simulink model "OPENXWD"  (R2022b)
settings: Solver=ode45  StartTime=0.0  StopTime=inf  RelTol=1e-3  EnableMultiTasking=on
PreLoadFcn:
  | run('Parameters\FSE_Parameters.m')
model workspace (MAT data in the model file):
  socvcb : containers.Map (value not decoded)
undefined symbols (not defined in the file): i_Diff
libraries: CarMaker4SL x21, simulink x16, eeGeneralControl x6
(part 3 of 8)

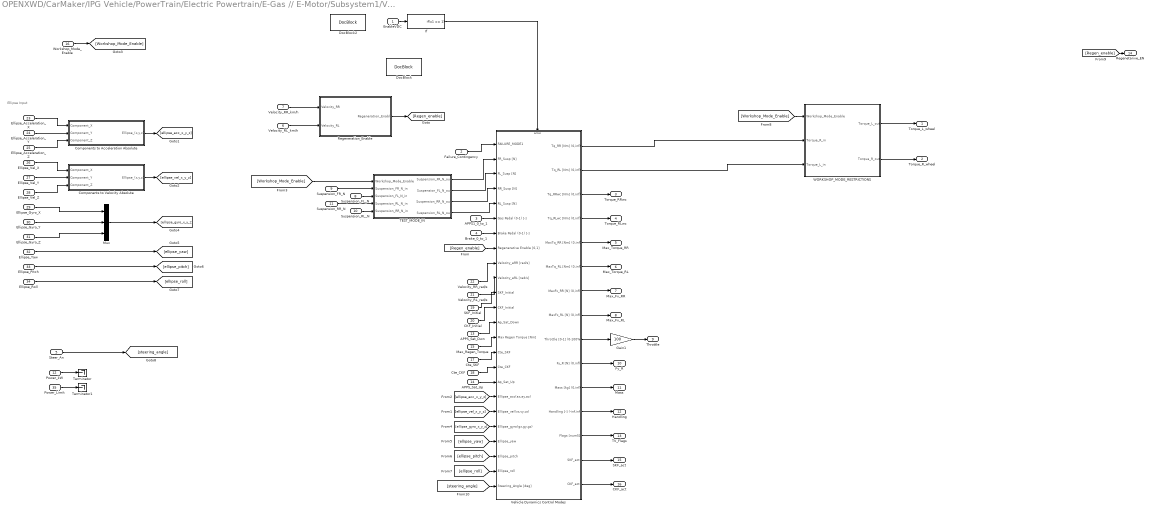
== system OPENXWD/CarMaker/IPG Vehicle/PowerTrain/Electric Powertrain/E-Gas // E-Motor/Subsystem1/VDC ==
  note: Ellipse Input
  EnableVDC : Inport
  Failure_Contingency : Inport  Port=2
  APPS1_0_to_1 : Inport  Port=3
  Brake_0_to_1 : Inport  Port=4
  Steer_An : Inport  Port=5
  Velocity_RL_km/h : Inport  Port=6
  Velocity_RR_km/h : Inport  Port=7
  Suspension_FL_N : Inport  Port=8
  Suspension_FR_N : Inport  Port=9
  Suspension_RL_N : Inport  Port=10
  Suspension_RR_N : Inport  Port=11
  Power_kW : Inport  Port=12
  APPS_Sat_Dwn : Inport  Port=13
  APPS_Sat_Up : Inport  Port=14
  Max_Regen_Torque : Inport  Port=15
  Workshop_Mode_Enable : Inport  Port=16
  Cte_SKF : Inport  Port=17
  Cte_CKF : Inport  Port=18
  SKF_Initial : Inport  Port=19
  CKF_Initial : Inport  Port=20
  Velocity_RL_rad/s : Inport  Port=21
  Velocity_RR_rad/s : Inport  Port=22
  Ellipse_Acceleration_X : Inport  Port=23
  Ellipse_Acceleration_Y : Inport  Port=24
  Ellipse_Acceleration_Z : Inport  Port=25
  Ellipse_Vel_X : Inport  Port=26
  Ellipse_Vel_Y : Inport  Port=27
  Ellipse_Vel_Z : Inport  Port=28
  Ellipse_Gyro_X : Inport  Port=29
  Ellipse_Gyro_Y : Inport  Port=30
  Ellipse_Gyro_Z : Inport  Port=31
  Ellipse_Yaw : Inport  Port=32
  Ellipse_Pitch : Inport  Port=33
  Ellipse_Roll : Inport  Port=34
  Power_Limit : Inport  Port=35
  Components to Acceleration Absolute : Subsystem
  Components to Velocity Absolute : Subsystem
  DocBlock : simulink/Model-Wide Utilities/DocBlock  DocumentType=Text
      content=|
      | This port activates the different modes that the VDC must be in according
      | to the signals that the Main ECU has available.
      |
      | Port Must be 1 to activate VDC 2018 Complete (Green)
      | Requirement: All sensors are connected (Ellipse, Steering, SuspensionRear
      | [SuspensionFront only needed to calculate Mass]).
      |
      | Port Must be 2 to activate VDC without Longitudinal (Yellow)
      | Requirement: No steering sensor data
      |
      | Port Must be 3 to activate Steering TV 2017 without TC (Orange)
      | Requirement: (No Ellipse) or (No SuspensionRear Data)
      |
      | Port Must be 4 to activate Rigid Axle (Red)
      | Requirement: (No Steering Sensor) and (No Ellipse or No SuspensionRear)
  DocBlock2 : simulink/Model-Wide Utilities/DocBlock  DocumentType=Text
      content=|
      | Enable Vehicle Dynamics Control.
      |
      | This port must be 1 if the calculations for VDC must be made
  Gain1 : Gain  Gain=100
  If : If  IfExpression=u1 == 1  ShowElse=off
  Mux : Mux  Inputs=3
  Regeneration_Enable : Subsystem  TreatAsAtomicUnit=on
  TEST_MODE_IN : Subsystem  TreatAsAtomicUnit=on
  Terminator : Terminator
  Terminator1 : Terminator
  Vehicle Dynamics Control Modes : Subsystem
  WORKSHOP_MODE_RESTRICTIONS : Subsystem  TreatAsAtomicUnit=on
  Torque_L_wheel : Outport  VectorParamsAs1DForOutWhenUnconnected=off
  Torque_R_wheel : Outport  Port=2  VectorParamsAs1DForOutWhenUnconnected=off
  Torque_RRwc : Outport  Port=3  VectorParamsAs1DForOutWhenUnconnected=off
  Torque_RLwc : Outport  Port=4  VectorParamsAs1DForOutWhenUnconnected=off
  Max_Torque_RR : Outport  Port=5  VectorParamsAs1DForOutWhenUnconnected=off
  Max_Torque_RL : Outport  Port=6  VectorParamsAs1DForOutWhenUnconnected=off
  Max_Fx_RR : Outport  Port=7  VectorParamsAs1DForOutWhenUnconnected=off
  Max_Fx_RL : Outport  Port=8  VectorParamsAs1DForOutWhenUnconnected=off
  Throttle : Outport  Port=9  VectorParamsAs1DForOutWhenUnconnected=off
  Fy_R : Outport  Port=10  VectorParamsAs1DForOutWhenUnconnected=off
  Mass : Outport  Port=11  VectorParamsAs1DForOutWhenUnconnected=off
  Handling : Outport  Port=12  VectorParamsAs1DForOutWhenUnconnected=off
  TV_Flags : Outport  Port=13  VectorParamsAs1DForOutWhenUnconnected=off
  Regenetarive_EN : Outport  Port=14  VectorParamsAs1DForOutWhenUnconnected=off
  SKF_act : Outport  Port=15  VectorParamsAs1DForOutWhenUnconnected=off
  CKF_act : Outport  Port=16  VectorParamsAs1DForOutWhenUnconnected=off
  wires:
  Velocity_RR_km/h/1 -> Regeneration_Enable/1(Velocity_RR)
  Gain1/1 -> Throttle/1
  Vehicle Dynamics Control Modes/7(MaxFx_RR [N] (0,inf)) -> Max_Fx_RR/1
  Vehicle Dynamics Control Modes/6(MaxTq_RL [Nm] (0,inf)) -> Max_Torque_RL/1
  Vehicle Dynamics Control Modes/8(MaxFx_RL [N] (0,inf)) -> Max_Fx_RL/1
  Power_kW/1 -> Terminator/1
  Vehicle Dynamics Control Modes/1(Tq_RR [Nm] (0,inf)) -> WORKSHOP_MODE_RESTRICTIONS/2(Torque_R_in)
  APPS_Sat_Up/1 -> Vehicle Dynamics Control Modes/17(Ap_Sat_Up)
  WORKSHOP_MODE_RESTRICTIONS/1(Torque_L_out) -> Torque_L_wheel/1
  Vehicle Dynamics Control Modes/3(Tq_RRwc [Nm] (0,inf)) -> Torque_RRwc/1
  Suspension_FL_N/1 -> TEST_MODE_IN/3(Suspension_FL_N_in)
  Suspension_FR_N/1 -> TEST_MODE_IN/2(Suspension_FR_N_in)
  TEST_MODE_IN/1(Suspension_FR_N_out) -> Vehicle Dynamics Control Modes/2(FR_Susp [N])
  Velocity_RR_rad/s/1 -> Vehicle Dynamics Control Modes/9(Velocity_eRR [rad/s])
  Vehicle Dynamics Control Modes/14(SKF_act) -> SKF_act/1
  APPS1_0_to_1/1 -> Vehicle Dynamics Control Modes/6(Gas Pedal (0-1) [-])
  Vehicle Dynamics Control Modes/4(Tq_RLwc [Nm] (0,inf)) -> Torque_RLwc/1
  Vehicle Dynamics Control Modes/5(MaxTq_RR [Nm] (0,inf)) -> Max_Torque_RR/1
  Brake_0_to_1/1 -> Vehicle Dynamics Control Modes/7(Brake Pedal (0-1) [-])
  Velocity_RL_km/h/1 -> Regeneration_Enable/2(Velocity_RL)
  Vehicle Dynamics Control Modes/11(Mass [kg] (0,inf)) -> Mass/1
  Vehicle Dynamics Control Modes/9(Throttle [0-1] (0-100%)) -> Gain1/1
  Vehicle Dynamics Control Modes/2(Tq_RL [Nm] (0,inf)) -> WORKSHOP_MODE_RESTRICTIONS/3(Torque_L_in)
  EnableVDC/1 -> If/1
  Suspension_RL_N/1 -> TEST_MODE_IN/5(Suspension_RR_N_in)
  Vehicle Dynamics Control Modes/10(Fy_R [N] (0,inf)) -> Fy_R/1
  Vehicle Dynamics Control Modes/13(Flags [num5]) -> TV_Flags/1
  [Workshop_Mode_Enable] -> TEST_MODE_IN/1(Workshop_Mode_Enable)
  Suspension_RR_N/1 -> TEST_MODE_IN/4(Suspension_RL_N_in)
  Vehicle Dynamics Control Modes/12(Handling [-] (-inf,inf)) -> Handling/1
  Workshop_Mode_Enable/1 -> [Workshop_Mode_Enable]
  Vehicle Dynamics Control Modes/15(CKF_act) -> CKF_act/1
  If/1 -> Vehicle Dynamics Control Modes/Action
  TEST_MODE_IN/2(Suspension_FL_N_out) -> Vehicle Dynamics Control Modes/3(FL_Susp [N])
  TEST_MODE_IN/3(Suspension_RR_N_out) -> Vehicle Dynamics Control Modes/4(RR_Susp [N])
  TEST_MODE_IN/4(Suspension_RL_N_out) -> Vehicle Dynamics Control Modes/5(RL_Susp [N])
  Velocity_RL_rad/s/1 -> Vehicle Dynamics Control Modes/10(Velocity_eRL [rad/s])
  SKF_Initial/1 -> Vehicle Dynamics Control Modes/11(SKF_Initial)
  CKF_Initial/1 -> Vehicle Dynamics Control Modes/12(CKF_Initial)
  APPS_Sat_Dwn/1 -> Vehicle Dynamics Control Modes/13(Ap_Sat_Down)
  Max_Regen_Torque/1 -> Vehicle Dynamics Control Modes/14(Max Regen Torque [Nm])
  Cte_SKF/1 -> Vehicle Dynamics Control Modes/15(Cte_SKF)
  Cte_CKF/1 -> Vehicle Dynamics Control Modes/16(Cte_CKF)
  Failure_Contingency/1 -> Vehicle Dynamics Control Modes/1(FAILURE_MODE1)
  Regeneration_Enable/1(Regeneration_Enable) -> [Regen_enable]
  [Regen_enable] -> Vehicle Dynamics Control Modes/8(Regenerative Enable [0,1])
  WORKSHOP_MODE_RESTRICTIONS/2(Torque_R_out) -> Torque_R_wheel/1
  Components to Acceleration Absolute/1(Ellipse_(x,y,z)) -> [ellipse_acc_x_y_z]
  Ellipse_Acceleration_X/1 -> Components to Acceleration Absolute/1(Component_X)
  Ellipse_Acceleration_Y/1 -> Components to Acceleration Absolute/2(Component_Y)
  Ellipse_Acceleration_Z/1 -> Components to Acceleration Absolute/3(Component_Z)
  Components to Velocity Absolute/1(Ellipse_(x,y,z)) -> [ellipse_vel_x_y_z]
  Ellipse_Vel_X/1 -> Components to Velocity Absolute/1(Component_X)
  Ellipse_Vel_Z/1 -> Components to Velocity Absolute/3(Component_Z)
  Ellipse_Vel_Y/1 -> Components to Velocity Absolute/2(Component_Y)
  Ellipse_Gyro_X/1 -> Mux/1
  Ellipse_Gyro_Y/1 -> Mux/2
  Ellipse_Gyro_Z/1 -> Mux/3
  Mux/1 -> [ellipse_gyro_x_y_z]
  Ellipse_Yaw/1 -> [ellipse_yaw]
  Ellipse_Pitch/1 -> [ellipse_pitch]
  Ellipse_Roll/1 -> [ellipse_roll]
  [ellipse_vel_x_y_z] -> Vehicle Dynamics Control Modes/19(Ellipse_vel(vx,vy,vz))
  [ellipse_acc_x_y_z] -> Vehicle Dynamics Control Modes/18(Ellipse_acc(ax,ay,az))
  [ellipse_gyro_x_y_z] -> Vehicle Dynamics Control Modes/20(Ellipse_gyro(gx,gy,gz))
  [ellipse_yaw] -> Vehicle Dynamics Control Modes/21(Ellipse_yaw)
  [ellipse_pitch] -> Vehicle Dynamics Control Modes/22(Ellipse_pitch)
  [ellipse_roll] -> Vehicle Dynamics Control Modes/23(Ellipse_roll)
  [Workshop_Mode_Enable] -> WORKSHOP_MODE_RESTRICTIONS/1(Workshop_Mode_Enable)
  [Regen_enable] -> Regenetarive_EN/1
  Steer_An/1 -> [steering_angle]
  [steering_angle] -> Vehicle Dynamics Control Modes/24(Steering_Angle [deg])
  Power_Limit/1 -> Terminator1/1

== system OPENXWD/CarMaker/IPG Vehicle/PowerTrain/Electric Powertrain/E-Gas // E-Motor/Subsystem1/W to kW ==
  Power : Inport
  0-100 to 0-2 : Constant  Value=1000
  Divide5 : Product  Inputs=*/
  Out : Outport  VectorParamsAs1DForOutWhenUnconnected=off
  wires:
  Power/1 -> Divide5/1
  0-100 to 0-2/1 -> Divide5/2
  Divide5/1 -> Out/1

== system OPENXWD/CarMaker/IPG Vehicle/PowerTrain/Electric Powertrain/E-Gas // E-Motor/Subsystem1/power_limitation ==
  note: Inputs:
      | max_cell_temp: signal from AMS_Master (Highest_Cell_Temp) [ºC]
      | max_inverter_temp: highest temperature of any of the inverters [ºC]
      | max_motor_temp: highest temperature of any of the motors [ºC]
      | SoC_Low, SoC_High: Lowest & Highest cell state of charge (0-100) [%]
  note: Outputs:
      | Flags: 1 means power is being limited by temperature, 0 means not limited
      | SoP_discharge: State of Power for discharging
      | SoP_charge: State of Power for charging
  max_motor_temp : Inport
  max_inverter_temp : Inport  Port=2
  max_cell_temp : Inport  Port=3
  SoC_Low : Inport  Port=4
  SoC_High : Inport  Port=5
  Saturation : Saturate  UpperLimit=1  LowerLimit=0
  Saturation1 : Saturate  UpperLimit=1  LowerLimit=0
  SoC_SoP : Subsystem
  initial_limitation : Constant  Value=0.4
  temperature_SoP : Subsystem
  Accu_Temperature_Limitation_Flag : Outport
  Inverters_Temperature_Limitation_Flag : Outport  Port=2
  Motors_Temperature_Limitation_Flag : Outport  Port=3
  SoP_Discharge : Outport  Port=4
  SoP_Regen : Outport  Port=5
  wires:
  SoC_SoP/1(SoP_Discharge) -> Saturation/1  "SoP_Discharge"
  SoC_SoP/2(SoP_Regen) -> Saturation1/1  "SoP_Regen"
  max_motor_temp/1 -> temperature_SoP/1(max_motor_temp)
  max_inverter_temp/1 -> temperature_SoP/2(max_inverter_temp)
  max_cell_temp/1 -> temperature_SoP/3(max_cell_temp), SoC_SoP/4(max_cell_temp)
  initial_limitation/1 -> temperature_SoP/4(initial_limitation)
  temperature_SoP/1(SoP) -> SoC_SoP/3(SoP_Temperature)  "temperature_SoP"
  temperature_SoP/4(Motors_Temperature_Limitation_Flag) -> Motors_Temperature_Limitation_Flag/1
  temperature_SoP/3(Inverters_Temperature_Limitation_Flag) -> Inverters_Temperature_Limitation_Flag/1
  temperature_SoP/2(Accu_Temperature_Limitation_Flag) -> Accu_Temperature_Limitation_Flag/1
  SoC_High/1 -> SoC_SoP/2(SoC_High)
  SoC_Low/1 -> SoC_SoP/1(SoC_Low)
  Saturation/1 -> SoP_Discharge/1
  Saturation1/1 -> SoP_Regen/1

== system OPENXWD/CarMaker/IPG Vehicle/PowerTrain/Electric Powertrain/E-Gas // E-Motor/Subsystem1/Accumulator Power/PowerLimitDetection ==
  note: mean:500ms
      | time:25ms
      | moving window: 500/25=20
  Power : Inport
  Data Store Memory10 : DataStoreMemory  ReadBeforeWriteMsg=warning  WriteAfterWriteMsg=warning  WriteAfterReadMsg=warning  ShowAdditionalParam=off
  Data Store Read30 : DataStoreRead  IndexOptions=Index vector (dialog)  Indices=1  OutputSizes=1
  Data Store Write20 : DataStoreWrite  IndexOptions=Index vector (dialog)  Indices=1  OutputSizes=1
  If : If  IfExpression=u1 >= 80000
  LimitReached : Subsystem  TreatAsAtomicUnit=on
  Merge1 : Merge
  OK_OrLatch : Subsystem  TreatAsAtomicUnit=on
  PowerLimitReached : Outport  VectorParamsAs1DForOutWhenUnconnected=off
  PowerMean500ms : Outport  Port=2  VectorParamsAs1DForOutWhenUnconnected=off
  wires:
  Power/1 -> If/1, PowerMean500ms/1
  If/1 -> LimitReached/Action
  If/2 -> OK_OrLatch/Action
  LimitReached/1("Out ") -> Merge1/1
  OK_OrLatch/1(Out 1) -> Merge1/2
  Merge1/1 -> Data Store Write20/1, PowerLimitReached/1
  Data Store Read30/1 -> OK_OrLatch/1(IN)

== system OPENXWD/CarMaker/IPG Vehicle/PowerTrain/Electric Powertrain/E-Gas // E-Motor/Subsystem1/Calculate Current Conversion/KT_L_TORKY ==
  Torque : Inport
  A/Nm : Gain  Gain=0.2
  Current : Outport  VectorParamsAs1DForOutWhenUnconnected=off
  wires:
  A/Nm/1 -> Current/1
  Torque/1 -> A/Nm/1

== system OPENXWD/CarMaker/IPG Vehicle/PowerTrain/Electric Powertrain/E-Gas // E-Motor/Subsystem1/Calculate Current Conversion/KT_R_EMY ==
  Torque : Inport
  A/Nm : Gain  Gain=0.2
  Current : Outport  VectorParamsAs1DForOutWhenUnconnected=off
  wires:
  Torque/1 -> A/Nm/1
  A/Nm/1 -> Current/1

== system OPENXWD/CarMaker/IPG Vehicle/PowerTrain/Electric Powertrain/E-Gas // E-Motor/Subsystem1/Controls Temperature by limiting Torque/SoC_SoP ==
  note: El lookup se puede obtener ensayando una celda en una descarga y en una carga con pérdidas de calor constantes. La corriente normalizada será el lookup.
  note: Si está descargada, no descargues más
  note: Si está cargada, no
      | cargues más
  SoC_Low : Inport
  SoC_High : Inport  Port=2
  SoP_Temperature : Inport  Port=3
  max_cell_temp : Inport  Port=4
  Gain5 : Gain  Gain=1/100
  Gain6 : Gain  Gain=1/100
  Lookup_SoC_SoP_chg : Lookup_n-D  NumberOfTableDimensions=1  BreakpointsForDimension1=[0.02 0.1 0.2 0.3 0.5 0.8 0.95 1]  Table=[0.95 1 1 1 1 0.9 0.75 0.02]  InternalRulePriority=Speed  RndMeth=Simplest
  Lookup_SoC_SoP_dischg : Lookup_n-D  NumberOfTableDimensions=1  BreakpointsForDimension1=[0.02 0.1 0.2 0.3 0.5 0.8 0.9 1]  Table=[0.4 0.6 0.8 0.95 1 1 0.98 0.95]  InternalRulePriority=Speed  RndMeth=Simplest
  Lookup_Temp_SoP_chg : Lookup_n-D  NumberOfTableDimensions=1  BreakpointsForDimension1=[45 48 49 50 51]  Table=[1 0.75 0.5 0 0]  InternalRulePriority=Speed  RndMeth=Simplest
  Product : Product
  Product4 : Product
  Product5 : Product
  SoP_Discharge : Outport
  SoP_Regen : Outport  Port=2
  wires:
  Lookup_SoC_SoP_dischg/1 -> Product4/1
  Product/1 -> Product5/2
  SoP_Temperature/1 -> Product4/2, Product5/1
  SoC_Low/1 -> Gain6/1
  Gain6/1 -> Lookup_SoC_SoP_dischg/1
  SoC_High/1 -> Gain5/1
  Gain5/1 -> Lookup_SoC_SoP_chg/1
  Product5/1 -> SoP_Regen/1
  Product4/1 -> SoP_Discharge/1
  Lookup_SoC_SoP_chg/1 -> Product/1
  max_cell_temp/1 -> Lookup_Temp_SoP_chg/1
  Lookup_Temp_SoP_chg/1 -> Product/2

== system OPENXWD/CarMaker/IPG Vehicle/PowerTrain/Electric Powertrain/E-Gas // E-Motor/Subsystem1/Controls Temperature by limiting Torque/temperature_SoP ==
  max_motor_temp : Inport
  max_inverter_temp : Inport  Port=2
  max_cell_temp : Inport  Port=3
  initial_limitation : Inport  Port=4
  Flag_Accu : simulink/Logic and Bit Operations/Compare To Constant  relop=<  const=1  OutDataTypeStr=boolean  ZeroCross=off
  Flag_Inv : simulink/Logic and Bit Operations/Compare To Constant  relop=<  const=1  OutDataTypeStr=boolean  ZeroCross=off
  Flag_Mot : simulink/Logic and Bit Operations/Compare To Constant  relop=<  const=1  OutDataTypeStr=boolean  ZeroCross=off
  Min : MinMax  Inputs=3
  temperature_rise_limitator_Accu : Subsystem
  temperature_rise_limitator_Inverters : Subsystem
  temperature_rise_limitator_Motors : Subsystem
  SoP : Outport
  Accu_Temperature_Limitation_Flag : Outport  Port=2
  Inverters_Temperature_Limitation_Flag : Outport  Port=3
  Motors_Temperature_Limitation_Flag : Outport  Port=4
  wires:
  temperature_rise_limitator_Inverters/1(SoP) -> Flag_Inv/1, Min/2
  initial_limitation/1 -> temperature_rise_limitator_Accu/2(initial_limitation), temperature_rise_limitator_Motors/2(initial_limitation), temperature_rise_limitator_Inverters/2(initial_limitation)
  Flag_Accu/1 -> Accu_Temperature_Limitation_Flag/1
  temperature_rise_limitator_Motors/1(SoP) -> Flag_Mot/1, Min/3
  max_cell_temp/1 -> temperature_rise_limitator_Accu/1(max_cell_temp)
  temperature_rise_limitator_Accu/1(SoP) -> Flag_Accu/1, Min/1
  Min/1 -> SoP/1
  Flag_Inv/1 -> Inverters_Temperature_Limitation_Flag/1
  Flag_Mot/1 -> Motors_Temperature_Limitation_Flag/1
  max_inverter_temp/1 -> temperature_rise_limitator_Inverters/1(max_inverter_temp)
  max_motor_temp/1 -> temperature_rise_limitator_Motors/1(max_motor_temp)

== system OPENXWD/CarMaker/IPG Vehicle/PowerTrain/Electric Powertrain/E-Gas // E-Motor/Subsystem1/SAFETY BLOCK/APPS_IMPLAUSIBILITY ==
  APPS1 : Inport
  APPS2 : Inport  Port=2
  Ab : Abs  SaturateOnIntegerOverflow=off
  If : If  IfExpression=u1 > 0.1
  Imp : Subsystem  TreatAsAtomicUnit=on
  Merge : Merge
  Not Imp : Subsystem  TreatAsAtomicUnit=on
  Sum : Sum  Inputs=|+-
  OK : Outport  VectorParamsAs1DForOutWhenUnconnected=off
  wires:
  APPS1/1 -> Sum/1
  APPS2/1 -> Sum/2
  Sum/1 -> Ab/1
  Ab/1 -> If/1
  Imp/1(Out1) -> Merge/1  "Bool 0"
  Not Imp/1(Out1) -> Merge/2  "Bool 1"
  Merge/1 -> OK/1
  If/2 -> Not Imp/Action
  If/1 -> Imp/Action

== system OPENXWD/CarMaker/IPG Vehicle/PowerTrain/Electric Powertrain/E-Gas // E-Motor/Subsystem1/VDC/Components to Acceleration Absolute ==
  Component_X : Inport
  Component_Y : Inport  Port=2
  Component_Z : Inport  Port=3
  Abs : Abs  SaturateOnIntegerOverflow=off
  Mux : Mux  Inputs=3
  Ellipse_(x,y,z) : Outport
  wires:
  Abs/1 -> Ellipse_(x,y,z)/1
  Component_Z/1 -> Mux/3
  Component_Y/1 -> Mux/2
  Mux/1 -> Abs/1
  Component_X/1 -> Mux/1

== system OPENXWD/CarMaker/IPG Vehicle/PowerTrain/Electric Powertrain/E-Gas // E-Motor/Subsystem1/VDC/Components to Velocity Absolute ==
  Component_X : Inport
  Component_Y : Inport  Port=2
  Component_Z : Inport  Port=3
  Abs : Abs  SaturateOnIntegerOverflow=off
  Mux : Mux  Inputs=3
  Ellipse_(x,y,z) : Outport
  wires:
  Abs/1 -> Ellipse_(x,y,z)/1
  Component_Z/1 -> Mux/3
  Component_Y/1 -> Mux/2
  Mux/1 -> Abs/1
  Component_X/1 -> Mux/1

== system OPENXWD/CarMaker/IPG Vehicle/PowerTrain/Electric Powertrain/E-Gas // E-Motor/Subsystem1/VDC/Regeneration_Enable ==
  note: Regen is Enable if velocity is higher than 2 km/h, to avoid backwards velocity due to Regen Tq (negative)
  Velocity_RR : Inport
  Velocity_RL : Inport  Port=2
  Enabled : Constant
  "Enabled " : Subsystem  TreatAsAtomicUnit=on
  If : If  NumInputs=2  IfExpression=(u1>2)&(u2>2)
  Merge1 : Merge
  NotEnabled : Subsystem  TreatAsAtomicUnit=on
  "Zero " : Constant  Value=0
  Regeneration_Enable : Outport  VectorParamsAs1DForOutWhenUnconnected=off
  wires:
  Merge1/1 -> Regeneration_Enable/1
  Velocity_RR/1 -> If/1
  Velocity_RL/1 -> If/2
  If/1 -> "Enabled "/Action
  If/2 -> NotEnabled/Action
  "Zero "/1 -> NotEnabled/1(In1)
  NotEnabled/1(Out1) -> Merge1/2
  "Enabled "/1(Out1) -> Merge1/1
  Enabled/1 -> "Enabled "/1(In1)

== system OPENXWD/CarMaker/IPG Vehicle/PowerTrain/Electric Powertrain/E-Gas // E-Motor/Subsystem1/VDC/TEST_MODE_IN ==
  Workshop_Mode_Enable : Inport
  Suspension_FR_N_in : Inport  Port=2
  Suspension_FL_N_in : Inport  Port=3
  Suspension_RL_N_in : Inport  Port=4
  Suspension_RR_N_in : Inport  Port=5
  BYPASS : Subsystem  TreatAsAtomicUnit=on
  If : If  IfExpression=u1 == 1
  Merge{,1..3} (4 alike) : Merge
  TEST_CONSTANTS : Subsystem  TreatAsAtomicUnit=on
  Suspension_FR_N_out : Outport  VectorParamsAs1DForOutWhenUnconnected=off
  Suspension_FL_N_out : Outport  Port=2  VectorParamsAs1DForOutWhenUnconnected=off
  Suspension_RR_N_out : Outport  Port=3  VectorParamsAs1DForOutWhenUnconnected=off
  Suspension_RL_N_out : Outport  Port=4  VectorParamsAs1DForOutWhenUnconnected=off
  wires:
  Suspension_FR_N_in/1 -> BYPASS/1(In1)
  Suspension_FL_N_in/1 -> BYPASS/2(In2)
  Suspension_RR_N_in/1 -> BYPASS/3(In3)
  Suspension_RL_N_in/1 -> BYPASS/4(In4)
  Merge/1 -> Suspension_FR_N_out/1
  Merge1/1 -> Suspension_FL_N_out/1
  Merge2/1 -> Suspension_RR_N_out/1
  Merge3/1 -> Suspension_RL_N_out/1
  BYPASS/1(Out1) -> Merge/1
  BYPASS/2(Out2) -> Merge1/1
  BYPASS/3(Out3) -> Merge2/1
  BYPASS/4(Out4) -> Merge3/1
  Workshop_Mode_Enable/1 -> If/1
  If/2 -> BYPASS/Action
  If/1 -> TEST_CONSTANTS/Action
  TEST_CONSTANTS/4(Out4) -> Merge3/2
  TEST_CONSTANTS/3(Out3) -> Merge2/2
  TEST_CONSTANTS/2(Out2) -> Merge1/2
  TEST_CONSTANTS/1(Out1) -> Merge/2

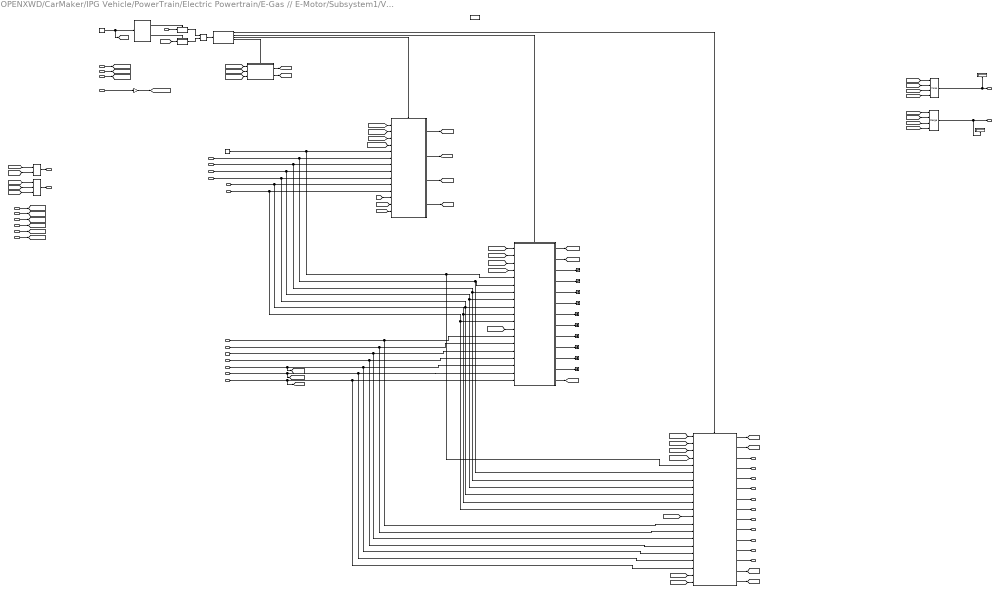
== system OPENXWD/CarMaker/IPG Vehicle/PowerTrain/Electric Powertrain/E-Gas // E-Motor/Subsystem1/VDC/Vehicle Dynamics Control Modes ==
  note: Handling now is negligible is always 0
  note: Ellipse Inputs
  note: Failure Mode Selection: 5 -> Automatic Failure Mode Selection according to sensors available
      | 4 -> Rigid Axle (red)
      | 3 -> Steering TV with TC (orange)
      | 2 -> VDC without longitudinal (yellow)
      | 1 -> VDC complete (green)
      | 0 -> TV with TC 2023
  FAILURE_MODE1 : Inport
  FR_Susp [N] : Inport  Port=2
  FL_Susp [N] : Inport  Port=3
  RR_Susp [N] : Inport  Port=4
  RL_Susp [N] : Inport  Port=5
  Gas Pedal (0-1) [-] : Inport  Port=6
  Brake Pedal (0-1) [-] : Inport  Port=7
  Regenerative Enable [0,1] : Inport  Port=8
  Velocity_eRR [rad/s] : Inport  Port=9
  Velocity_eRL [rad/s] : Inport  Port=10
  SKF_Initial : Inport  Port=11
  CKF_Initial : Inport  Port=12
  Ap_Sat_Down : Inport  Port=13
  Max Regen Torque [Nm] : Inport  Port=14
  Cte_SKF : Inport  Port=15
  Cte_CKF : Inport  Port=16
  Ap_Sat_Up : Inport  Port=17
  Ellipse_acc(ax,ay,az) : Inport  Port=18
  Ellipse_vel(vx,vy,vz) : Inport  Port=19
  Ellipse_gyro(gx,gy,gz) : Inport  Port=20
  Ellipse_yaw : Inport  Port=21
  Ellipse_pitch : Inport  Port=22
  Ellipse_roll : Inport  Port=23
  Steering_Angle [deg] : Inport  Port=24
  Action Port : ActionPort  ActionPortLabel=if(u1 == 1)
  Automatic Failure Mode : Subsystem  TreatAsAtomicUnit=on
  Constant : Constant  Value=5
  Display : Display
  Display1 : Display
  FAILURE MODE : If  IfExpression=u1 == 1  ElseIfExpressions=u1 == 2, u1 == 3, u1 == 4, u1 == 0  ShowElse=off
  Gain : Gain  Gain=-1
  If : If  IfExpression=u1 == 5
  Manual Failure Mode Selection : Subsystem  TreatAsAtomicUnit=on
  Merge : Merge
  Merge Tq_RL : Merge  Inputs=4
  Merge Tq_RR : Merge  Inputs=4
  Merge2 : Merge
  Merge3 : Merge  Inputs=3
  Rigid Axle : Subsystem  TreatAsAtomicUnit=on
  Steering TV with TC : Subsystem  TreatAsAtomicUnit=on
  "Steering Wheel Saturation (per site) [deg] " : Constant  Value=10
  Terminator{,1..9} (10 alike) : Terminator
  VDC Complete : Subsystem  TreatAsAtomicUnit=on
  VDC without Longitudinal : Subsystem  TreatAsAtomicUnit=on
  Tq_RR [Nm] (0,inf) : Outport  VectorParamsAs1DForOutWhenUnconnected=off
  Tq_RL [Nm] (0,inf) : Outport  Port=2  VectorParamsAs1DForOutWhenUnconnected=off
  Tq_RRwc [Nm] (0,inf) : Outport  Port=3  VectorParamsAs1DForOutWhenUnconnected=off
  Tq_RLwc [Nm] (0,inf) : Outport  Port=4  VectorParamsAs1DForOutWhenUnconnected=off
  MaxTq_RR [Nm] (0,inf) : Outport  Port=5  VectorParamsAs1DForOutWhenUnconnected=off
  MaxTq_RL [Nm] (0,inf) : Outport  Port=6  VectorParamsAs1DForOutWhenUnconnected=off
  MaxFx_RR [N] (0,inf) : Outport  Port=7  VectorParamsAs1DForOutWhenUnconnected=off
  MaxFx_RL [N] (0,inf) : Outport  Port=8  VectorParamsAs1DForOutWhenUnconnected=off
  Throttle [0-1] (0-100%) : Outport  Port=9  VectorParamsAs1DForOutWhenUnconnected=off
  Fy_R [N] (0,inf) : Outport  Port=10  VectorParamsAs1DForOutWhenUnconnected=off
  Mass [kg] (0,inf) : Outport  Port=11  VectorParamsAs1DForOutWhenUnconnected=off
  Handling [-] (-inf,inf) : Outport  Port=12  VectorParamsAs1DForOutWhenUnconnected=off
  Flags [num5] : Outport  Port=13  VectorParamsAs1DForOutWhenUnconnected=off
  SKF_act : Outport  Port=14  VectorParamsAs1DForOutWhenUnconnected=off
  CKF_act : Outport  Port=15  VectorParamsAs1DForOutWhenUnconnected=off
  wires:
  VDC Complete/4(Tq_RLwc [Nm] (0,inf)) -> Tq_RLwc [Nm] (0,inf)/1
  VDC Complete/3(Tq_RRwc [Nm] (0,inf)) -> Tq_RRwc [Nm] (0,inf)/1
  VDC Complete/5(MaxTq_RR [Nm] (0,inf)) -> MaxTq_RR [Nm] (0,inf)/1
  VDC Complete/6(MaxTq_RL [Nm] (0,inf)) -> MaxTq_RL [Nm] (0,inf)/1
  VDC Complete/7(MaxFx_RR [N] (0,inf)) -> MaxFx_RR [N] (0,inf)/1
  VDC Complete/8(MaxFx_RL [N] (0,inf)) -> MaxFx_RL [N] (0,inf)/1
  VDC Complete/9(Throttle [0-1] (0-100%)) -> Throttle [0-1] (0-100%)/1
  VDC Complete/10(Fy_R [N] (0,inf)) -> Fy_R [N] (0,inf)/1
  VDC Complete/11(Mass [kg] (0,inf)) -> Mass [kg] (0,inf)/1
  VDC Complete/12(Handling [-] (-inf,inf)) -> Handling [-] (-inf,inf)/1
  VDC without Longitudinal/3(MaxTq_RR [Nm] (0,inf)) -> Terminator/1
  VDC without Longitudinal/4(MaxTq_RL [Nm] (0,inf)) -> Terminator1/1
  VDC without Longitudinal/5(MaxFx_RR [N] (0,inf)) -> Terminator2/1
  VDC without Longitudinal/6(MaxFx_RL [N] (0,inf)) -> Terminator3/1
  VDC without Longitudinal/7(Fy_R [N] (0,inf)) -> Terminator4/1
  VDC without Longitudinal/8(Throttle [0-1] (0-100%)) -> Terminator5/1
  VDC without Longitudinal/9(Mass [kg] (0,inf)) -> Terminator6/1
  VDC without Longitudinal/10(Handling [-] (-inf,inf)) -> Terminator7/1
  VDC without Longitudinal/11(Tq_RRwc [Nm] (0,inf)) -> Terminator8/1
  VDC without Longitudinal/12(Tq_RLwc [Nm] (0,inf)) -> Terminator9/1
  VDC Complete/13(Flags_[num5]) -> Flags [num5]/1
  Merge2/1 -> SKF_act/1
  Merge3/1 -> CKF_act/1
  "Steering Wheel Saturation (per site) [deg] "/1 -> Steering TV with TC/5("Steering Wheel Saturation (per site) "), VDC without Longitudinal/5(Steering Saturation (per site) [deg]), VDC Complete/5(Steering Saturation (per site) [deg])
  SKF_Initial/1 -> VDC without Longitudinal/6(SKF_initial), VDC Complete/6(SKF_Initial), Steering TV with TC/6(SKF_Initial)
  CKF_Initial/1 -> VDC Complete/7(CKF_Initial), VDC without Longitudinal/7(CKF_Initial), Steering TV with TC/7(CKF_Initial)
  Cte_SKF/1 -> VDC Complete/8(Cte_SKF), VDC without Longitudinal/8(Cte_SKF), Steering TV with TC/8(Cte_SKF)
  Cte_CKF/1 -> VDC Complete/9(Cte_CKF), VDC without Longitudinal/9(Cte_CKF), Steering TV with TC/9(Cte_CKF)
  Velocity_eRL [rad/s]/1 -> Steering TV with TC/10(Vel_eRL), VDC Complete/10(Velocity_eRL [rad/s]), VDC without Longitudinal/10(Velocity_eRL [rad/s])
  Velocity_eRR [rad/s]/1 -> Steering TV with TC/11(Vel_eRR), VDC Complete/11(Velocity_eRR [rad/s]), VDC without Longitudinal/11(Velocity_eRR [rad/s])
  Steering TV with TC/3(SKF_act) -> [SKF_act2]
  Steering TV with TC/4(CKF_act) -> [CKF_act2]
  VDC without Longitudinal/13(CKF_act) -> [CKF_act1]
  VDC Complete/14(SKF_act) -> [SKF_act0]
  VDC Complete/15(CKF_act) -> [CKF_act0]
  [CKF_act1] -> Merge3/2
  [CKF_act0] -> Merge3/1
  [CKF_act2] -> Merge3/3
  [SKF_act0] -> Merge2/1
  [SKF_act2] -> Merge2/2
  FAILURE MODE/1 -> VDC Complete/Action
  FAILURE MODE/2 -> VDC without Longitudinal/Action
  FAILURE MODE/3 -> Steering TV with TC/Action
  FAILURE MODE/4 -> Rigid Axle/Action
  Brake Pedal (0-1) [-]/1 -> VDC Complete/19(Brake Pedal (0-1) [-]), VDC without Longitudinal/19(Brake Pedal (0-1) [-]), [Bp]
  FR_Susp [N]/1 -> VDC Complete/13(FR_Susp [N]), VDC without Longitudinal/13(FR_Susp [N])
  FL_Susp [N]/1 -> VDC Complete/14(FL_Susp [N]), VDC without Longitudinal/14(FL_Susp [N])
  RR_Susp [N]/1 -> VDC Complete/15(RR_Susp [N]), VDC without Longitudinal/15(RR_Susp [N])
  RL_Susp [N]/1 -> VDC Complete/16(RL_Susp [N]), VDC without Longitudinal/16(RL_Susp [N])
  Regenerative Enable [0,1]/1 -> [Regen_enable], VDC Complete/17(Regenerative Enable [0,1]), VDC without Longitudinal/17(Regenerative Enable [0,1])
  Max Regen Torque [Nm]/1 -> [Max_Regen_Tq], VDC Complete/18(Max Regen Torque [Nm]), VDC without Longitudinal/18(Max Regen Torque [Nm])
  Steering TV with TC/1(Tq_RR_E2 [Nm] (0,inf)) -> [Tq_RR_E2]
  Steering TV with TC/2(Tq_RL_E2 [Nm] (0,inf)) -> [Tq_RL_E2]
  VDC without Longitudinal/1(Tq_RR_E1 [Nm] (0,inf)) -> [Tq_RR_E1]
  VDC Complete/1(Tq_RR_E0 [Nm] (0,inf)) -> [Tq_RR_E0]
  VDC Complete/2(Tq_RL_E0 [Nm] (0,inf)) -> [Tq_RL_E0]
  Merge Tq_RR/1 -> Display/1, Tq_RR [Nm] (0,inf)/1
  Rigid Axle/1(Tq_RR_E3 [Nm] (0,inf)) -> [Tq_RR_E3]
  Rigid Axle/2(Tq_RL_E3 [Nm] (0,inf)) -> [Tq_RL_E3]
  Merge Tq_RL/1 -> Display1/1, Tq_RL [Nm] (0,inf)/1
  [Tq_RR_E0] -> Merge Tq_RR/4
  [Tq_RR_E1] -> Merge Tq_RR/3
  [Tq_RR_E2] -> Merge Tq_RR/2
  [Tq_RR_E3] -> Merge Tq_RR/1
  [Tq_RL_E0] -> Merge Tq_RL/4
  [Tq_RL_E1] -> Merge Tq_RL/3
  [Tq_RL_E2] -> Merge Tq_RL/2
  [Tq_RL_E3] -> Merge Tq_RL/1
  [Bp] -> Steering TV with TC/12(Bp)
  [Max_Regen_Tq] -> Steering TV with TC/13(Max_Regen_Tq)
  [Regen_enable] -> Steering TV with TC/14(Regen_enable)
  If/1 -> Automatic Failure Mode/Action
  FAILURE_MODE1/1 -> Automatic Failure Mode/1(In1)
  If/2 -> Manual Failure Mode Selection/Action
  Constant/1 -> [FM_select], If/1
  [FM_select] -> Manual Failure Mode Selection/1(In1)
  Merge/1 -> FAILURE MODE/1
  Automatic Failure Mode/1(Out1) -> Merge/1
  Manual Failure Mode Selection/1(Out1) -> Merge/2
  VDC without Longitudinal/2(Tq_RL_E1 [Nm] (0,inf)) -> [Tq_RL_E1]
  Ellipse_acc(ax,ay,az)/1 -> [ellipse_acc_ax_ay_az]
  Ellipse_vel(vx,vy,vz)/1 -> [ellipse_vel_vx_vy_vz]
  Ellipse_gyro(gx,gy,gz)/1 -> [ellipse_gyro_gx_gy_gz]
  Ellipse_yaw/1 -> [ellipse_yaw]
  Ellipse_pitch/1 -> [ellipse_pitch]
  Ellipse_roll/1 -> [ellipse_roll]
  [ellipse_acc_ax_ay_az] -> VDC without Longitudinal/12(Ellipse_acc_ax_ay_az)
  [ellipse_acc_ax_ay_az] -> VDC Complete/12(Ellipse_acc)
  [ellipse_gyro_gx_gy_gz] -> VDC Complete/20(Gyro_Ellipse)
  [ellipse_vel_vx_vy_vz] -> VDC Complete/21(Ellipse_vel)
  Gas Pedal (0-1) [-]/1 -> [gas_pedal_0_1]
  [gas_pedal_0_1] -> Rigid Axle/3(Gas Pedal [0-1])
  [gas_pedal_0_1] -> Steering TV with TC/3(Gas Pedal [0-1])
  [gas_pedal_0_1] -> VDC without Longitudinal/3(Gas Pedal (0-1) [-])
  [gas_pedal_0_1] -> VDC Complete/3(Gas Pedal (0-1) [-])
  Ap_Sat_Up/1 -> [ap_sat_up]
  Ap_Sat_Down/1 -> [ap_sat_down]
  [ap_sat_up] -> Rigid Axle/1("Ap_Sat_up ")
  [ap_sat_down] -> Rigid Axle/2(Ap_Sat_down)
  [ap_sat_up] -> Steering TV with TC/1("Ap_Sat_up ")
  [ap_sat_down] -> Steering TV with TC/2(Ap_Sat_down)
  [ap_sat_up] -> VDC without Longitudinal/1(Ap_Sat_Up [-])
  [ap_sat_down] -> VDC without Longitudinal/2(Ap_Sat_Down [-])
  [ap_sat_down] -> VDC Complete/2(Ap_Sat_Down [-])
  [ap_sat_up] -> VDC Complete/1(Ap_Sat_Up [-])
  Steering_Angle [deg]/1 -> Gain/1
  Gain/1 -> [steering_angle_normalized]
  [steering_angle_normalized] -> Steering TV with TC/4(Steering_Angle [deg])
  [steering_angle_normalized] -> VDC without Longitudinal/4(Steering_Angle [deg])
  [steering_angle_normalized] -> VDC Complete/4(Steering_Angle [deg])

== system OPENXWD/CarMaker/IPG Vehicle/PowerTrain/Electric Powertrain/E-Gas // E-Motor/Subsystem1/VDC/WORKSHOP_MODE_RESTRICTIONS ==
  Workshop_Mode_Enable : Inport
  Torque_R_in : Inport  Port=2
  Torque_L_in : Inport  Port=3
  BYPASS : Subsystem  TreatAsAtomicUnit=on
  If : If  IfExpression=u1 == 1
  Merge : Merge
  Merge1 : Merge
  Saturation : Saturate  UpperLimit=580  LowerLimit=-580
  Saturation1 : Saturate  UpperLimit=580  LowerLimit=-580
  "Torque_Reduction " : Subsystem  TreatAsAtomicUnit=on
  Torque_L_out : Outport  VectorParamsAs1DForOutWhenUnconnected=off
  Torque_R_out : Outport  Port=2  VectorParamsAs1DForOutWhenUnconnected=off
  wires:
  If/2 -> BYPASS/Action
  If/1 -> "Torque_Reduction "/Action
  Workshop_Mode_Enable/1 -> If/1
  Torque_R_in/1 -> "Torque_Reduction "/1(In1), BYPASS/1(In1)
  Torque_L_in/1 -> "Torque_Reduction "/2(In2), BYPASS/2(In2)
  BYPASS/1(Out1) -> Merge/1
  BYPASS/2(Out2) -> Merge1/2
  "Torque_Reduction "/1(Out1) -> Merge/2
  "Torque_Reduction "/2(Out2) -> Merge1/1
  Merge/1 -> Saturation/1
  Merge1/1 -> Saturation1/1
  Saturation/1 -> Torque_R_out/1
  Saturation1/1 -> Torque_L_out/1

== system OPENXWD/CarMaker/IPG Vehicle/PowerTrain/Electric Powertrain/E-Gas // E-Motor/Subsystem1/power_limitation/SoC_SoP ==
  note: El lookup se puede obtener ensayando una celda en una descarga y en una carga con pérdidas de calor constantes. La corriente normalizada será el lookup.
  note: Si está descargada, no descargues más
  note: Si está cargada, no
      | cargues más
  SoC_Low : Inport
  SoC_High : Inport  Port=2
  SoP_Temperature : Inport  Port=3
  max_cell_temp : Inport  Port=4
  Gain5 : Gain  Gain=1/100
  Gain6 : Gain  Gain=1/100
  Lookup_SoC_SoP_chg : Lookup_n-D  NumberOfTableDimensions=1  BreakpointsForDimension1=[0.02 0.1 0.2 0.3 0.5 0.8 0.95 1]  Table=[0.95 1 1 1 1 0.9 0.75 0.02]  InternalRulePriority=Speed  RndMeth=Simplest
  Lookup_SoC_SoP_dischg : Lookup_n-D  NumberOfTableDimensions=1  BreakpointsForDimension1=[0.02 0.1 0.2 0.3 0.5 0.8 0.9 1]  Table=[0.4 0.6 0.8 0.95 1 1 0.98 0.95]  InternalRulePriority=Speed  RndMeth=Simplest
  Lookup_Temp_SoP_chg : Lookup_n-D  NumberOfTableDimensions=1  BreakpointsForDimension1=[45 48 49 50 51]  Table=[1 0.75 0.5 0 0]  InternalRulePriority=Speed  RndMeth=Simplest
  Product : Product
  Product4 : Product
  Product5 : Product
  SoP_Discharge : Outport
  SoP_Regen : Outport  Port=2
  wires:
  Lookup_SoC_SoP_dischg/1 -> Product4/1
  Product/1 -> Product5/2
  SoP_Temperature/1 -> Product4/2, Product5/1
  SoC_Low/1 -> Gain6/1
  Gain6/1 -> Lookup_SoC_SoP_dischg/1
  SoC_High/1 -> Gain5/1
  Gain5/1 -> Lookup_SoC_SoP_chg/1
  Product5/1 -> SoP_Regen/1
  Product4/1 -> SoP_Discharge/1
  Lookup_SoC_SoP_chg/1 -> Product/1
  max_cell_temp/1 -> Lookup_Temp_SoP_chg/1
  Lookup_Temp_SoP_chg/1 -> Product/2

== system OPENXWD/CarMaker/IPG Vehicle/PowerTrain/Electric Powertrain/E-Gas // E-Motor/Subsystem1/power_limitation/temperature_SoP ==
  max_motor_temp : Inport
  max_inverter_temp : Inport  Port=2
  max_cell_temp : Inport  Port=3
  initial_limitation : Inport  Port=4
  Flag_Accu : simulink/Logic and Bit Operations/Compare To Constant  relop=<  const=1  OutDataTypeStr=boolean  ZeroCross=off
  Flag_Inv : simulink/Logic and Bit Operations/Compare To Constant  relop=<  const=1  OutDataTypeStr=boolean  ZeroCross=off
  Flag_Mot : simulink/Logic and Bit Operations/Compare To Constant  relop=<  const=1  OutDataTypeStr=boolean  ZeroCross=off
  Min : MinMax  Inputs=3
  temperature_rise_limitator_Accu : Subsystem
  temperature_rise_limitator_Inverters : Subsystem
  temperature_rise_limitator_Motors : Subsystem
  SoP : Outport
  Accu_Temperature_Limitation_Flag : Outport  Port=2
  Inverters_Temperature_Limitation_Flag : Outport  Port=3
  Motors_Temperature_Limitation_Flag : Outport  Port=4
  wires:
  temperature_rise_limitator_Inverters/1(SoP) -> Flag_Inv/1, Min/2
  initial_limitation/1 -> temperature_rise_limitator_Accu/2(initial_limitation), temperature_rise_limitator_Motors/2(initial_limitation), temperature_rise_limitator_Inverters/2(initial_limitation)
  Flag_Accu/1 -> Accu_Temperature_Limitation_Flag/1
  temperature_rise_limitator_Motors/1(SoP) -> Flag_Mot/1, Min/3
  max_cell_temp/1 -> temperature_rise_limitator_Accu/1(max_cell_temp)
  temperature_rise_limitator_Accu/1(SoP) -> Flag_Accu/1, Min/1
  Min/1 -> SoP/1
  Flag_Inv/1 -> Inverters_Temperature_Limitation_Flag/1
  Flag_Mot/1 -> Motors_Temperature_Limitation_Flag/1
  max_inverter_temp/1 -> temperature_rise_limitator_Inverters/1(max_inverter_temp)
  max_motor_temp/1 -> temperature_rise_limitator_Motors/1(max_motor_temp)

== system OPENXWD/CarMaker/IPG Vehicle/PowerTrain/Electric Powertrain/E-Gas // E-Motor/Subsystem1/Accumulator Power/PowerLimitDetection/LimitReached ==
  Action Port : ActionPort  ActionPortLabel=if(u1 >= 80000)
  Constant : Constant
  "Out " : Outport  VectorParamsAs1DForOutWhenUnconnected=off
  wires:
  Constant/1 -> "Out "/1

== system OPENXWD/CarMaker/IPG Vehicle/PowerTrain/Electric Powertrain/E-Gas // E-Motor/Subsystem1/Accumulator Power/PowerLimitDetection/OK_OrLatch ==
  IN : Inport
  Action Port : ActionPort  ActionPortLabel=else
  If : If  IfExpression=(u1>0)
  Latched Error : Subsystem  TreatAsAtomicUnit=on
  Merge : Merge
  OK : Subsystem  TreatAsAtomicUnit=on
  Out 1 : Outport  VectorParamsAs1DForOutWhenUnconnected=off
  wires:
  IN/1 -> If/1
  If/1 -> Latched Error/Action
  If/2 -> OK/Action
  Latched Error/1("Out ") -> Merge/1
  OK/1("Out ") -> Merge/2
  Merge/1 -> Out 1/1

== system OPENXWD/CarMaker/IPG Vehicle/PowerTrain/Electric Powertrain/E-Gas // E-Motor/Subsystem1/Controls Temperature by limiting Torque/temperature_SoP/temperature_rise_limitator_Accu ==
  note: initial_limitation es una constante para la reducción inicial (de 0 a 1, más bajo significa que cambia
      | menos, más alto la limitación
      | inicial es más bestia).
  note: saturamos de 1 a 0 por si acaso
  note: magia chunga para
      | que los números cuadren
  note: Se limita la corriente en proporción
      | al ratio entre la temperatura actual y 50ºC
  note: output 0 si está por
      | debajo de 50ºC, 1 si está
      | por encima
  max_cell_temp : Inport
  initial_limitation : Inport  Port=2
  Add1 : Sum  Inputs=-+
  Add2 : Sum  Inputs=-++
  Add3 : Sum  Inputs=+-
  Constant1 : Constant  Value=45
  Constant2 : Constant  Value=5
  Constant3 : Constant
  Divide : Product  Inputs=*/
  Low-Pass Filter (Discrete or Continuous)1 : eeGeneralControl/Low-Pass Filter (Discrete or Continuous)  K=1  T=100  B=inf  A=-inf  init_option=Inherited from block input  x0=0  Ts=-1
  Product4 : Product
  Saturation1 : Saturate  UpperLimit=1  LowerLimit=0
  Temp higher than 50 : simulink/Logic and Bit Operations/Compare To Constant  relop=>=  const=50  OutDataTypeStr=boolean  ZeroCross=off
  SoP : Outport
  wires:
  Divide/1 -> Add3/1
  Constant3/1 -> Add2/3
  Constant1/1 -> Divide/1
  max_cell_temp/1 -> Add1/2, Temp higher than 50/1
  Temp higher than 50/1 -> Add2/1, Product4/2
  Constant2/1 -> Add1/1
  Product4/1 -> Add2/2
  Add2/1 -> Low-Pass Filter (Discrete or Continuous)1/1
  Add3/1 -> Product4/1
  Add1/1 -> Divide/2
  Saturation1/1 -> SoP/1
  initial_limitation/1 -> Add3/2
  Low-Pass Filter (Discrete or Continuous)1/1 -> Saturation1/1

== system OPENXWD/CarMaker/IPG Vehicle/PowerTrain/Electric Powertrain/E-Gas // E-Motor/Subsystem1/Controls Temperature by limiting Torque/temperature_SoP/temperature_rise_limitator_Inverters ==
  note: output 0 si está por
      | debajo de 50ºC, 1 si está
      | por encima
  note: Se limita la corriente en proporción
      | al ratio entre la temperatura actual y 50ºC
  note: magia chunga para
      | que los números cuadren
  note: saturamos de 1 a 0 por si acaso
  note: initial_limitation es una constante para la reducción inicial (de 0 a 1, más bajo significa que cambia
      | menos, más alto la limitación
      | inicial es más bestia).
  max_inverter_temp : Inport
  initial_limitation : Inport  Port=2
  Add1 : Sum  Inputs=-+
  Add2 : Sum  Inputs=-++
  Add3 : Sum  Inputs=+-
  Constant1 : Constant  Value=45
  Constant2 : Constant  Value=5
  Constant3 : Constant
  Divide : Product  Inputs=*/
  Low-Pass Filter (Discrete or Continuous) : eeGeneralControl/Low-Pass Filter (Discrete or Continuous)  K=1  T=100  B=inf  A=-inf  init_option=Inherited from block input  x0=0  Ts=-1
  Product4 : Product
  Saturation1 : Saturate  UpperLimit=1  LowerLimit=0
  Temp higher than 50 : simulink/Logic and Bit Operations/Compare To Constant  relop=>=  const=50  OutDataTypeStr=boolean  ZeroCross=off
  SoP : Outport
  wires:
  Low-Pass Filter (Discrete or Continuous)/1 -> Saturation1/1
  initial_limitation/1 -> Add3/2
  Saturation1/1 -> SoP/1
  Add1/1 -> Divide/2
  Add3/1 -> Product4/1
  Add2/1 -> Low-Pass Filter (Discrete or Continuous)/1
  Product4/1 -> Add2/2
  Constant2/1 -> Add1/1
  Temp higher than 50/1 -> Product4/2, Add2/1
  max_inverter_temp/1 -> Temp higher than 50/1, Add1/2
  Constant1/1 -> Divide/1
  Constant3/1 -> Add2/3
  Divide/1 -> Add3/1

== system OPENXWD/CarMaker/IPG Vehicle/PowerTrain/Electric Powertrain/E-Gas // E-Motor/Subsystem1/Controls Temperature by limiting Torque/temperature_SoP/temperature_rise_limitator_Motors ==
  note: initial_limitation es una constante para la reducción inicial (de 0 a 1, más bajo significa que cambia
      | menos, más alto la limitación
      | inicial es más bestia).
  note: saturamos de 1 a 0 por si acaso
  note: magia chunga para
      | que los números cuadren
  note: Se limita la corriente en proporción
      | al ratio entre la temperatura actual y 110ºC
  note: output 0 si está por
      | debajo de 110ºC, 1 si está
      | por encima
  max_motor_temp : Inport
  initial_limitation : Inport  Port=2
  Add1 : Sum  Inputs=-+
  Add2 : Sum  Inputs=-++
  Add3 : Sum  Inputs=+-
  Constant1 : Constant  Value=105
  Constant2 : Constant  Value=5
  Constant3 : Constant
  Divide : Product  Inputs=*/
  Low-Pass Filter (Discrete or Continuous) : eeGeneralControl/Low-Pass Filter (Discrete or Continuous)  K=1  T=100  B=inf  A=-inf  init_option=Inherited from block input  x0=0  Ts=-1
  Product4 : Product
  Saturation1 : Saturate  UpperLimit=1  LowerLimit=0
  Temp higher than 110 : simulink/Logic and Bit Operations/Compare To Constant  relop=>=  const=110  OutDataTypeStr=boolean  ZeroCross=off
  SoP : Outport
  wires:
  Divide/1 -> Add3/1
  Constant3/1 -> Add2/3
  Constant1/1 -> Divide/1
  max_motor_temp/1 -> Add1/2, Temp higher than 110/1
  Temp higher than 110/1 -> Add2/1, Product4/2
  Constant2/1 -> Add1/1
  Product4/1 -> Add2/2
  Add2/1 -> Low-Pass Filter (Discrete or Continuous)/1
  Add3/1 -> Product4/1
  Add1/1 -> Divide/2
  Saturation1/1 -> SoP/1
  initial_limitation/1 -> Add3/2
  Low-Pass Filter (Discrete or Continuous)/1 -> Saturation1/1

== system OPENXWD/CarMaker/IPG Vehicle/PowerTrain/Electric Powertrain/E-Gas // E-Motor/Subsystem1/SAFETY BLOCK/APPS_IMPLAUSIBILITY/Imp ==
  Action Port : ActionPort  ActionPortLabel=if(u1 > 0.1)
  Constant : Constant  Value=0  OutDataTypeStr=boolean
  Out1 : Outport  VectorParamsAs1DForOutWhenUnconnected=off
  wires:
  Constant/1 -> Out1/1  "Boolean"

== system OPENXWD/CarMaker/IPG Vehicle/PowerTrain/Electric Powertrain/E-Gas // E-Motor/Subsystem1/SAFETY BLOCK/APPS_IMPLAUSIBILITY/Not Imp ==
  Action Port : ActionPort  ActionPortLabel=else
  Constant : Constant  OutDataTypeStr=boolean
  Out1 : Outport  VectorParamsAs1DForOutWhenUnconnected=off
  wires:
  Constant/1 -> Out1/1  "Boolean"

== system OPENXWD/CarMaker/IPG Vehicle/PowerTrain/Electric Powertrain/E-Gas // E-Motor/Subsystem1/VDC/Regeneration_Enable/Enabled  ==
  In1 : Inport
  Action Port : ActionPort  ActionPortLabel=if((u1>2)&(u2>2))
  Out1 : Outport  VectorParamsAs1DForOutWhenUnconnected=off
  wires:
  In1/1 -> Out1/1

== system OPENXWD/CarMaker/IPG Vehicle/PowerTrain/Electric Powertrain/E-Gas // E-Motor/Subsystem1/VDC/Regeneration_Enable/NotEnabled ==
  In1 : Inport
  Action Port : ActionPort  ActionPortLabel=else
  Out1 : Outport  VectorParamsAs1DForOutWhenUnconnected=off
  wires:
  In1/1 -> Out1/1

== system OPENXWD/CarMaker/IPG Vehicle/PowerTrain/Electric Powertrain/E-Gas // E-Motor/Subsystem1/VDC/TEST_MODE_IN/BYPASS ==
  In1 : Inport
  In2 : Inport  Port=2
  In3 : Inport  Port=3
  In4 : Inport  Port=4
  Action Port : ActionPort  ActionPortLabel=else
  Out1 : Outport  VectorParamsAs1DForOutWhenUnconnected=off
  Out2 : Outport  Port=2  VectorParamsAs1DForOutWhenUnconnected=off
  Out3 : Outport  Port=3  VectorParamsAs1DForOutWhenUnconnected=off
  Out4 : Outport  Port=4  VectorParamsAs1DForOutWhenUnconnected=off
  wires:
  In1/1 -> Out1/1
  In2/1 -> Out2/1
  In3/1 -> Out3/1
  In4/1 -> Out4/1

== system OPENXWD/CarMaker/IPG Vehicle/PowerTrain/Electric Powertrain/E-Gas // E-Motor/Subsystem1/VDC/TEST_MODE_IN/TEST_CONSTANTS ==
  Action Port : ActionPort  ActionPortLabel=if(u1 == 1)
  Constant{,1..3} (4 alike) : Constant  Value=800
  Out1 : Outport  VectorParamsAs1DForOutWhenUnconnected=off
  Out2 : Outport  Port=2  VectorParamsAs1DForOutWhenUnconnected=off
  Out3 : Outport  Port=3  VectorParamsAs1DForOutWhenUnconnected=off
  Out4 : Outport  Port=4  VectorParamsAs1DForOutWhenUnconnected=off
  wires:
  Constant/1 -> Out1/1
  Constant1/1 -> Out2/1
  Constant2/1 -> Out3/1
  Constant3/1 -> Out4/1

== system OPENXWD/CarMaker/IPG Vehicle/PowerTrain/Electric Powertrain/E-Gas // E-Motor/Subsystem1/VDC/Vehicle Dynamics Control Modes/Automatic Failure Mode ==
  In1 : Inport
  Action Port : ActionPort  ActionPortLabel=if(u1 == 5)
  Out1 : Outport  VectorParamsAs1DForOutWhenUnconnected=off
  wires:
  In1/1 -> Out1/1

== system OPENXWD/CarMaker/IPG Vehicle/PowerTrain/Electric Powertrain/E-Gas // E-Motor/Subsystem1/VDC/Vehicle Dynamics Control Modes/Manual Failure Mode Selection ==
  In1 : Inport
  Action Port : ActionPort  ActionPortLabel=else
  Out1 : Outport  VectorParamsAs1DForOutWhenUnconnected=off
  wires:
  In1/1 -> Out1/1

== system OPENXWD/CarMaker/IPG Vehicle/PowerTrain/Electric Powertrain/E-Gas // E-Motor/Subsystem1/VDC/Vehicle Dynamics Control Modes/Rigid Axle ==
  "Ap_Sat_up " : Inport
  Ap_Sat_down : Inport  Port=2
  Gas Pedal [0-1] : Inport  Port=3
  Action Port : ActionPort  ActionPortLabel=elseif( u1 == 4)
  Accelerating : Subsystem
  RT_L : Gain  Gain=4
  RT_R : Gain  Gain=4
  Torque_RL [Nm] : Constant  Value=60
  Torque_RR [Nm] : Constant  Value=60
  Tq_RR_E3 [Nm] (0,inf) : Outport  VectorParamsAs1DForOutWhenUnconnected=off
  Tq_RL_E3 [Nm] (0,inf) : Outport  Port=2  VectorParamsAs1DForOutWhenUnconnected=off
  wires:
  Torque_RR [Nm]/1 -> RT_R/1
  Torque_RL [Nm]/1 -> RT_L/1
  Accelerating/2(Tq_RL) -> Tq_RL_E3 [Nm] (0,inf)/1
  Accelerating/1("Tq_RR ") -> Tq_RR_E3 [Nm] (0,inf)/1
  Gas Pedal [0-1]/1 -> Accelerating/1(Ap)
  "Ap_Sat_up "/1 -> Accelerating/2("Ap_Sat_up ")
  Ap_Sat_down/1 -> Accelerating/3(Ap_Sat_down)
  RT_R/1 -> Accelerating/4(Tq_RR)
  RT_L/1 -> Accelerating/5("Tq_RL ")

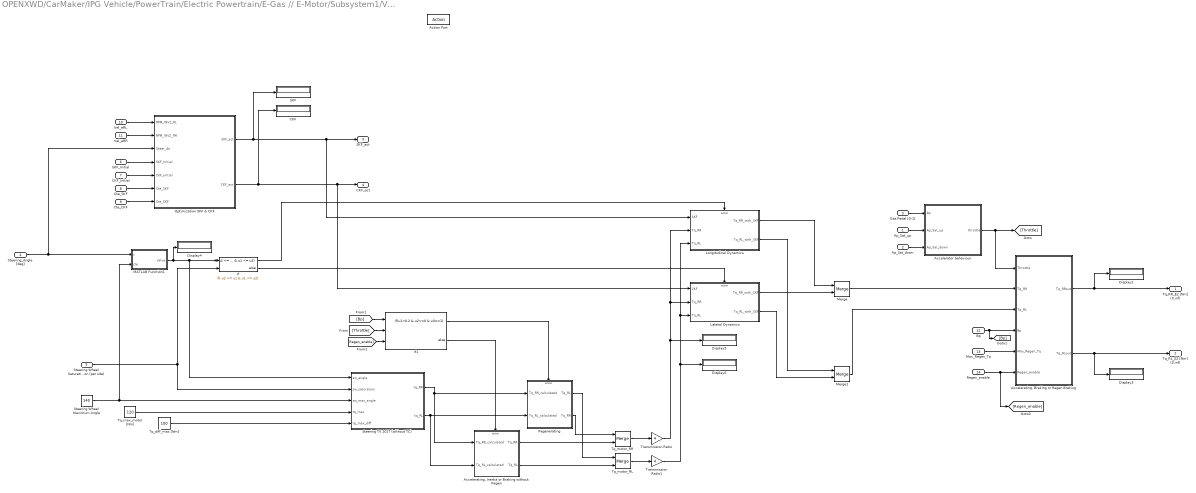
== system OPENXWD/CarMaker/IPG Vehicle/PowerTrain/Electric Powertrain/E-Gas // E-Motor/Subsystem1/VDC/Vehicle Dynamics Control Modes/Steering TV with TC ==
  "Ap_Sat_up " : Inport
  Ap_Sat_down : Inport  Port=2
  Gas Pedal [0-1] : Inport  Port=3
  Steering_Angle [deg] : Inport  Port=4
  "Steering Wheel Saturation (per site) " : Inport  Port=5
  SKF_Initial : Inport  Port=6
  CKF_Initial : Inport  Port=7
  Cte_SKF : Inport  Port=8
  Cte_CKF : Inport  Port=9
  Vel_eRL : Inport  Port=10
  Vel_eRR : Inport  Port=11
  Bp : Inport  Port=12
  Max_Regen_Tq : Inport  Port=13
  Regen_enable : Inport  Port=14
  Action Port : ActionPort  ActionPortLabel=elseif( u1 == 3)
  "Accelerating, Braking or Regen Braking" : Subsystem
  "Accelerating, Inertia or Braking without Regen" : Subsystem  TreatAsAtomicUnit=on
  Accelerator behaviour : MATLAB Function  TreatAsAtomicUnit=on
  CKF : Display
  Display{2..6} (5 alike) : Display
  If : If  NumInputs=2  IfExpression=-u2 <= u1 & u1 <= u2
  If1 : If  NumInputs=3  IfExpression=u1>0.2 & u2<=0 & u3==1
  Lateral Dynamics : Subsystem  TreatAsAtomicUnit=on
  Longitudinal Dynamics : Subsystem  TreatAsAtomicUnit=on
  MATLAB Function1 : MATLAB Function  TreatAsAtomicUnit=on
  Merge : Merge
  Merge1 : Merge
  Optimization SKF & CKF : Subsystem
  Regenerating : Subsystem  TreatAsAtomicUnit=on
  SKF : Display
  Steering TV 2017 (without TC) : MATLAB Function  TreatAsAtomicUnit=on
  Steering Wheel Maximum Angle : Constant  Value=140
  Tq_diff_max [Nm] : Constant  Value=100
  Tq_max_motor [Nm] : Constant  Value=120
  Tq_motor_RL : Merge
  Tq_motor_RR : Merge
  Transmission Ratio : Gain  Gain=4
  Transmission Ratio1 : Gain  Gain=4
  Tq_RR_E2 [Nm] (0,inf) : Outport  VectorParamsAs1DForOutWhenUnconnected=off
  Tq_RL_E2 [Nm] (0,inf) : Outport  Port=2  VectorParamsAs1DForOutWhenUnconnected=off
  SKF_act : Outport  Port=3  VectorParamsAs1DForOutWhenUnconnected=off
  CKF_act : Outport  Port=4  VectorParamsAs1DForOutWhenUnconnected=off
  wires:
  Steering Wheel Maximum Angle/1 -> Steering TV 2017 (without TC)/3(sw_max_angle), MATLAB Function1/2(cte)
  "Steering Wheel Saturation (per site) "/1 -> Steering TV 2017 (without TC)/2(sw_saturation), If/2
  Transmission Ratio/1 -> Display5/1, Longitudinal Dynamics/2(Tq_RR), Lateral Dynamics/2(Tq_RR)
  Tq_motor_RL/1 -> Transmission Ratio1/1
  MATLAB Function1/1(value) -> Display4/1, Steering TV 2017 (without TC)/1(sw_angle), If/1
  Optimization SKF & CKF/2(CKF_act) -> CKF/1, Lateral Dynamics/1(CKF), CKF_act/1
  SKF_Initial/1 -> Optimization SKF & CKF/4(SKF_Initial)
  Cte_SKF/1 -> Optimization SKF & CKF/6(Cte_SKF)
  Vel_eRL/1 -> Optimization SKF & CKF/1(RPM_INV1_RL)
  Vel_eRR/1 -> Optimization SKF & CKF/2(RPM_INV2_RR)
  Optimization SKF & CKF/1(SKF_act) -> SKF_act/1, Longitudinal Dynamics/1(SKF), SKF/1
  Steering_Angle [deg]/1 -> MATLAB Function1/1(v), Optimization SKF & CKF/3(Steer_An)
  CKF_Initial/1 -> Optimization SKF & CKF/5(CKF_Initial)
  Cte_CKF/1 -> Optimization SKF & CKF/7(Cte_CKF)
  If/1 -> Longitudinal Dynamics/Action
  Lateral Dynamics/2(Tq_RL_with_CKF) -> Merge1/2
  If/2 -> Lateral Dynamics/Action
  Longitudinal Dynamics/2(Tq_RL_with_SKF) -> Merge1/1
  Longitudinal Dynamics/1(Tq_RR_with_SKF) -> Merge/1
  Lateral Dynamics/1(Tq_RR_with_CKF) -> Merge/2
  Merge/1 -> "Accelerating, Braking or Regen Braking"/2(Tq_RR)
  Merge1/1 -> "Accelerating, Braking or Regen Braking"/3("Tq_RL ")
  "Accelerating, Braking or Regen Braking"/1(Tq_RRout) -> Display2/1, Tq_RR_E2 [Nm] (0,inf)/1
  "Accelerating, Braking or Regen Braking"/2(Tq_RLout) -> Tq_RL_E2 [Nm] (0,inf)/1, Display3/1
  Bp/1 -> [Bp], "Accelerating, Braking or Regen Braking"/4(Bp)
  Max_Regen_Tq/1 -> "Accelerating, Braking or Regen Braking"/5(Max_Regen_Tq)
  Regen_enable/1 -> [Regen_enable], "Accelerating, Braking or Regen Braking"/6(Regen_enable)
  Gas Pedal [0-1]/1 -> Accelerator behaviour/1(Ap)
  "Ap_Sat_up "/1 -> Accelerator behaviour/2(Ap_Sat_up)
  Ap_Sat_down/1 -> Accelerator behaviour/3(Ap_Sat_down)
  Accelerator behaviour/1(throttle) -> [Throttle], "Accelerating, Braking or Regen Braking"/1(Throttle)
  [Throttle] -> If1/2
  [Bp] -> If1/1
  [Regen_enable] -> If1/3
  If1/1 -> Regenerating/Action
  If1/2 -> "Accelerating, Inertia or Braking without Regen"/Action
  Steering TV 2017 (without TC)/2(tq_RL) -> "Accelerating, Inertia or Braking without Regen"/2(Tq_RL_calculated), Regenerating/2(Tq_RL_calculated)
  Steering TV 2017 (without TC)/1(tq_RR) -> "Accelerating, Inertia or Braking without Regen"/1(Tq_RR_calculated), Regenerating/1(Tq_RR_calculated)
  Regenerating/2(Tq_RR) -> Tq_motor_RR/1
  "Accelerating, Inertia or Braking without Regen"/1(Tq_RR) -> Tq_motor_RR/2
  Regenerating/1(Tq_RL) -> Tq_motor_RL/1
  "Accelerating, Inertia or Braking without Regen"/2(Tq_RL) -> Tq_motor_RL/2
  Tq_max_motor [Nm]/1 -> Steering TV 2017 (without TC)/4(tq_max)
  Tq_diff_max [Nm]/1 -> Steering TV 2017 (without TC)/5(tq_max_diff)
  Tq_motor_RR/1 -> Transmission Ratio/1
  Transmission Ratio1/1 -> Display6/1, Longitudinal Dynamics/3(Tq_RL), Lateral Dynamics/3(Tq_RL)
